simulink model "c00015M_harness"  (R2018a)
settings: Solver=FixedStepAuto  StartTime=0.0  StopTime=300  FixedStep=0.1  RelTol=1e-3
undefined symbols (not defined in the file): A1, hmax, PriorityTank, R1, R2, sigbuilder_block, TempThreshold
(part 3 of 33)

== system c00015M_harness/Eval21 ==
  In1 : Inport
  In3 : Inport  Port=2
  Constant2 : Constant
  Data Type Conversion : DataTypeConversion
  Data Type Conversion2 : DataTypeConversion
  Memory1 : Memory  InitialCondition=1
  Memory3 : Memory  InitialCondition=1
  MinMax : MinMax  Inputs=3
  MinMax1 : MinMax  Inputs=2
  MinMax3 : MinMax  Inputs=2
  ROOut1 : RelationalOperator  Operator===  OutDataTypeStr=boolean  RndMeth=Simplest
  ROOut3 : RelationalOperator  Operator===  OutDataTypeStr=boolean  RndMeth=Simplest
  Out1 : Outport
  wires:
  Data Type Conversion2/1 -> MinMax3/1
  Data Type Conversion/1 -> MinMax1/1
  MinMax1/1 -> Memory1/1, MinMax/1
  ROOut1/1 -> Data Type Conversion/1
  Memory3/1 -> MinMax3/2
  ROOut3/1 -> Data Type Conversion2/1
  MinMax3/1 -> Memory3/1, MinMax/3
  Memory1/1 -> MinMax1/2
  In1/1 -> ROOut1/1
  [out1] -> ROOut1/2
  In3/1 -> ROOut3/1
  [out3] -> ROOut3/2
  MinMax/1 -> Out1/1
  Constant2/1 -> MinMax/2

== system c00015M_harness/Eval22 ==
  In1 : Inport
  In3 : Inport  Port=2
  Constant2 : Constant
  Data Type Conversion : DataTypeConversion
  Data Type Conversion2 : DataTypeConversion
  Memory1 : Memory  InitialCondition=1
  Memory3 : Memory  InitialCondition=1
  MinMax : MinMax  Inputs=3
  MinMax1 : MinMax  Inputs=2
  MinMax3 : MinMax  Inputs=2
  ROOut1 : RelationalOperator  Operator===  OutDataTypeStr=boolean  RndMeth=Simplest
  ROOut3 : RelationalOperator  Operator===  OutDataTypeStr=boolean  RndMeth=Simplest
  Out1 : Outport
  wires:
  Data Type Conversion2/1 -> MinMax3/1
  Data Type Conversion/1 -> MinMax1/1
  MinMax1/1 -> Memory1/1, MinMax/1
  ROOut1/1 -> Data Type Conversion/1
  Memory3/1 -> MinMax3/2
  ROOut3/1 -> Data Type Conversion2/1
  MinMax3/1 -> Memory3/1, MinMax/3
  Memory1/1 -> MinMax1/2
  In1/1 -> ROOut1/1
  [out1] -> ROOut1/2
  In3/1 -> ROOut3/1
  [out3] -> ROOut3/2
  MinMax/1 -> Out1/1
  Constant2/1 -> MinMax/2

== system c00015M_harness/Eval220 ==
  In1 : Inport
  In3 : Inport  Port=2
  Constant2 : Constant
  Data Type Conversion : DataTypeConversion
  Data Type Conversion2 : DataTypeConversion
  Memory1 : Memory  InitialCondition=1
  Memory3 : Memory  InitialCondition=1
  MinMax : MinMax  Inputs=3
  MinMax1 : MinMax  Inputs=2
  MinMax3 : MinMax  Inputs=2
  ROOut1 : RelationalOperator  Operator===  OutDataTypeStr=boolean  RndMeth=Simplest
  ROOut3 : RelationalOperator  Operator===  OutDataTypeStr=boolean  RndMeth=Simplest
  Out1 : Outport
  wires:
  Data Type Conversion2/1 -> MinMax3/1
  Data Type Conversion/1 -> MinMax1/1
  MinMax1/1 -> Memory1/1, MinMax/1
  ROOut1/1 -> Data Type Conversion/1
  Memory3/1 -> MinMax3/2
  ROOut3/1 -> Data Type Conversion2/1
  MinMax3/1 -> Memory3/1, MinMax/3
  Memory1/1 -> MinMax1/2
  In1/1 -> ROOut1/1
  [out1] -> ROOut1/2
  In3/1 -> ROOut3/1
  [out3] -> ROOut3/2
  MinMax/1 -> Out1/1
  Constant2/1 -> MinMax/2

== system c00015M_harness/Eval221 ==
  In1 : Inport
  In3 : Inport  Port=2
  Constant2 : Constant
  Data Type Conversion : DataTypeConversion
  Data Type Conversion2 : DataTypeConversion
  Memory1 : Memory  InitialCondition=1
  Memory3 : Memory  InitialCondition=1
  MinMax : MinMax  Inputs=3
  MinMax1 : MinMax  Inputs=2
  MinMax3 : MinMax  Inputs=2
  ROOut1 : RelationalOperator  Operator===  OutDataTypeStr=boolean  RndMeth=Simplest
  ROOut3 : RelationalOperator  Operator===  OutDataTypeStr=boolean  RndMeth=Simplest
  Out1 : Outport
  wires:
  Data Type Conversion2/1 -> MinMax3/1
  Data Type Conversion/1 -> MinMax1/1
  MinMax1/1 -> Memory1/1, MinMax/1
  ROOut1/1 -> Data Type Conversion/1
  Memory3/1 -> MinMax3/2
  ROOut3/1 -> Data Type Conversion2/1
  MinMax3/1 -> Memory3/1, MinMax/3
  Memory1/1 -> MinMax1/2
  In1/1 -> ROOut1/1
  [out1] -> ROOut1/2
  In3/1 -> ROOut3/1
  [out3] -> ROOut3/2
  MinMax/1 -> Out1/1
  Constant2/1 -> MinMax/2

== system c00015M_harness/Eval222 ==
  In1 : Inport
  In3 : Inport  Port=2
  Constant2 : Constant
  Data Type Conversion : DataTypeConversion
  Data Type Conversion2 : DataTypeConversion
  Memory1 : Memory  InitialCondition=1
  Memory3 : Memory  InitialCondition=1
  MinMax : MinMax  Inputs=3
  MinMax1 : MinMax  Inputs=2
  MinMax3 : MinMax  Inputs=2
  ROOut1 : RelationalOperator  Operator===  OutDataTypeStr=boolean  RndMeth=Simplest
  ROOut3 : RelationalOperator  Operator===  OutDataTypeStr=boolean  RndMeth=Simplest
  Out1 : Outport
  wires:
  Data Type Conversion2/1 -> MinMax3/1
  Data Type Conversion/1 -> MinMax1/1
  MinMax1/1 -> Memory1/1, MinMax/1
  ROOut1/1 -> Data Type Conversion/1
  Memory3/1 -> MinMax3/2
  ROOut3/1 -> Data Type Conversion2/1
  MinMax3/1 -> Memory3/1, MinMax/3
  Memory1/1 -> MinMax1/2
  In1/1 -> ROOut1/1
  [out1] -> ROOut1/2
  In3/1 -> ROOut3/1
  [out3] -> ROOut3/2
  MinMax/1 -> Out1/1
  Constant2/1 -> MinMax/2

== system c00015M_harness/Eval223 ==
  In1 : Inport
  In3 : Inport  Port=2
  Constant2 : Constant
  Data Type Conversion : DataTypeConversion
  Data Type Conversion2 : DataTypeConversion
  Memory1 : Memory  InitialCondition=1
  Memory3 : Memory  InitialCondition=1
  MinMax : MinMax  Inputs=3
  MinMax1 : MinMax  Inputs=2
  MinMax3 : MinMax  Inputs=2
  ROOut1 : RelationalOperator  Operator===  OutDataTypeStr=boolean  RndMeth=Simplest
  ROOut3 : RelationalOperator  Operator===  OutDataTypeStr=boolean  RndMeth=Simplest
  Out1 : Outport
  wires:
  Data Type Conversion2/1 -> MinMax3/1
  Data Type Conversion/1 -> MinMax1/1
  MinMax1/1 -> Memory1/1, MinMax/1
  ROOut1/1 -> Data Type Conversion/1
  Memory3/1 -> MinMax3/2
  ROOut3/1 -> Data Type Conversion2/1
  MinMax3/1 -> Memory3/1, MinMax/3
  Memory1/1 -> MinMax1/2
  In1/1 -> ROOut1/1
  [out1] -> ROOut1/2
  In3/1 -> ROOut3/1
  [out3] -> ROOut3/2
  MinMax/1 -> Out1/1
  Constant2/1 -> MinMax/2

== system c00015M_harness/Eval224 ==
  In1 : Inport
  In3 : Inport  Port=2
  Constant2 : Constant
  Data Type Conversion : DataTypeConversion
  Data Type Conversion2 : DataTypeConversion
  Memory1 : Memory  InitialCondition=1
  Memory3 : Memory  InitialCondition=1
  MinMax : MinMax  Inputs=3
  MinMax1 : MinMax  Inputs=2
  MinMax3 : MinMax  Inputs=2
  ROOut1 : RelationalOperator  Operator===  OutDataTypeStr=boolean  RndMeth=Simplest
  ROOut3 : RelationalOperator  Operator===  OutDataTypeStr=boolean  RndMeth=Simplest
  Out1 : Outport
  wires:
  Data Type Conversion2/1 -> MinMax3/1
  Data Type Conversion/1 -> MinMax1/1
  MinMax1/1 -> Memory1/1, MinMax/1
  ROOut1/1 -> Data Type Conversion/1
  Memory3/1 -> MinMax3/2
  ROOut3/1 -> Data Type Conversion2/1
  MinMax3/1 -> Memory3/1, MinMax/3
  Memory1/1 -> MinMax1/2
  In1/1 -> ROOut1/1
  [out1] -> ROOut1/2
  In3/1 -> ROOut3/1
  [out3] -> ROOut3/2
  MinMax/1 -> Out1/1
  Constant2/1 -> MinMax/2

== system c00015M_harness/Eval225 ==
  In1 : Inport
  In3 : Inport  Port=2
  Constant2 : Constant
  Data Type Conversion : DataTypeConversion
  Data Type Conversion2 : DataTypeConversion
  Memory1 : Memory  InitialCondition=1
  Memory3 : Memory  InitialCondition=1
  MinMax : MinMax  Inputs=3
  MinMax1 : MinMax  Inputs=2
  MinMax3 : MinMax  Inputs=2
  ROOut1 : RelationalOperator  Operator===  OutDataTypeStr=boolean  RndMeth=Simplest
  ROOut3 : RelationalOperator  Operator===  OutDataTypeStr=boolean  RndMeth=Simplest
  Out1 : Outport
  wires:
  Data Type Conversion2/1 -> MinMax3/1
  Data Type Conversion/1 -> MinMax1/1
  MinMax1/1 -> Memory1/1, MinMax/1
  ROOut1/1 -> Data Type Conversion/1
  Memory3/1 -> MinMax3/2
  ROOut3/1 -> Data Type Conversion2/1
  MinMax3/1 -> Memory3/1, MinMax/3
  Memory1/1 -> MinMax1/2
  In1/1 -> ROOut1/1
  [out1] -> ROOut1/2
  In3/1 -> ROOut3/1
  [out3] -> ROOut3/2
  MinMax/1 -> Out1/1
  Constant2/1 -> MinMax/2

== system c00015M_harness/Eval226 ==
  In1 : Inport
  In3 : Inport  Port=2
  Constant2 : Constant
  Data Type Conversion : DataTypeConversion
  Data Type Conversion2 : DataTypeConversion
  Memory1 : Memory  InitialCondition=1
  Memory3 : Memory  InitialCondition=1
  MinMax : MinMax  Inputs=3
  MinMax1 : MinMax  Inputs=2
  MinMax3 : MinMax  Inputs=2
  ROOut1 : RelationalOperator  Operator===  OutDataTypeStr=boolean  RndMeth=Simplest
  ROOut3 : RelationalOperator  Operator===  OutDataTypeStr=boolean  RndMeth=Simplest
  Out1 : Outport
  wires:
  Data Type Conversion2/1 -> MinMax3/1
  Data Type Conversion/1 -> MinMax1/1
  MinMax1/1 -> Memory1/1, MinMax/1
  ROOut1/1 -> Data Type Conversion/1
  Memory3/1 -> MinMax3/2
  ROOut3/1 -> Data Type Conversion2/1
  MinMax3/1 -> Memory3/1, MinMax/3
  Memory1/1 -> MinMax1/2
  In1/1 -> ROOut1/1
  [out1] -> ROOut1/2
  In3/1 -> ROOut3/1
  [out3] -> ROOut3/2
  MinMax/1 -> Out1/1
  Constant2/1 -> MinMax/2

== system c00015M_harness/Eval227 ==
  In1 : Inport
  In3 : Inport  Port=2
  Constant2 : Constant
  Data Type Conversion : DataTypeConversion
  Data Type Conversion2 : DataTypeConversion
  Memory1 : Memory  InitialCondition=1
  Memory3 : Memory  InitialCondition=1
  MinMax : MinMax  Inputs=3
  MinMax1 : MinMax  Inputs=2
  MinMax3 : MinMax  Inputs=2
  ROOut1 : RelationalOperator  Operator===  OutDataTypeStr=boolean  RndMeth=Simplest
  ROOut3 : RelationalOperator  Operator===  OutDataTypeStr=boolean  RndMeth=Simplest
  Out1 : Outport
  wires:
  Data Type Conversion2/1 -> MinMax3/1
  Data Type Conversion/1 -> MinMax1/1
  MinMax1/1 -> Memory1/1, MinMax/1
  ROOut1/1 -> Data Type Conversion/1
  Memory3/1 -> MinMax3/2
  ROOut3/1 -> Data Type Conversion2/1
  MinMax3/1 -> Memory3/1, MinMax/3
  Memory1/1 -> MinMax1/2
  In1/1 -> ROOut1/1
  [out1] -> ROOut1/2
  In3/1 -> ROOut3/1
  [out3] -> ROOut3/2
  MinMax/1 -> Out1/1
  Constant2/1 -> MinMax/2

== system c00015M_harness/Eval228 ==
  In1 : Inport
  In3 : Inport  Port=2
  Constant2 : Constant
  Data Type Conversion : DataTypeConversion
  Data Type Conversion2 : DataTypeConversion
  Memory1 : Memory  InitialCondition=1
  Memory3 : Memory  InitialCondition=1
  MinMax : MinMax  Inputs=3
  MinMax1 : MinMax  Inputs=2
  MinMax3 : MinMax  Inputs=2
  ROOut1 : RelationalOperator  Operator===  OutDataTypeStr=boolean  RndMeth=Simplest
  ROOut3 : RelationalOperator  Operator===  OutDataTypeStr=boolean  RndMeth=Simplest
  Out1 : Outport
  wires:
  Data Type Conversion2/1 -> MinMax3/1
  Data Type Conversion/1 -> MinMax1/1
  MinMax1/1 -> Memory1/1, MinMax/1
  ROOut1/1 -> Data Type Conversion/1
  Memory3/1 -> MinMax3/2
  ROOut3/1 -> Data Type Conversion2/1
  MinMax3/1 -> Memory3/1, MinMax/3
  Memory1/1 -> MinMax1/2
  In1/1 -> ROOut1/1
  [out1] -> ROOut1/2
  In3/1 -> ROOut3/1
  [out3] -> ROOut3/2
  MinMax/1 -> Out1/1
  Constant2/1 -> MinMax/2

== system c00015M_harness/Eval229 ==
  In1 : Inport
  In3 : Inport  Port=2
  Constant2 : Constant
  Data Type Conversion : DataTypeConversion
  Data Type Conversion2 : DataTypeConversion
  Memory1 : Memory  InitialCondition=1
  Memory3 : Memory  InitialCondition=1
  MinMax : MinMax  Inputs=3
  MinMax1 : MinMax  Inputs=2
  MinMax3 : MinMax  Inputs=2
  ROOut1 : RelationalOperator  Operator===  OutDataTypeStr=boolean  RndMeth=Simplest
  ROOut3 : RelationalOperator  Operator===  OutDataTypeStr=boolean  RndMeth=Simplest
  Out1 : Outport
  wires:
  Data Type Conversion2/1 -> MinMax3/1
  Data Type Conversion/1 -> MinMax1/1
  MinMax1/1 -> Memory1/1, MinMax/1
  ROOut1/1 -> Data Type Conversion/1
  Memory3/1 -> MinMax3/2
  ROOut3/1 -> Data Type Conversion2/1
  MinMax3/1 -> Memory3/1, MinMax/3
  Memory1/1 -> MinMax1/2
  In1/1 -> ROOut1/1
  [out1] -> ROOut1/2
  In3/1 -> ROOut3/1
  [out3] -> ROOut3/2
  MinMax/1 -> Out1/1
  Constant2/1 -> MinMax/2

== system c00015M_harness/Eval23 ==
  In1 : Inport
  In3 : Inport  Port=2
  Constant2 : Constant
  Data Type Conversion : DataTypeConversion
  Data Type Conversion2 : DataTypeConversion
  Memory1 : Memory  InitialCondition=1
  Memory3 : Memory  InitialCondition=1
  MinMax : MinMax  Inputs=3
  MinMax1 : MinMax  Inputs=2
  MinMax3 : MinMax  Inputs=2
  ROOut1 : RelationalOperator  Operator===  OutDataTypeStr=boolean  RndMeth=Simplest
  ROOut3 : RelationalOperator  Operator===  OutDataTypeStr=boolean  RndMeth=Simplest
  Out1 : Outport
  wires:
  Data Type Conversion2/1 -> MinMax3/1
  Data Type Conversion/1 -> MinMax1/1
  MinMax1/1 -> Memory1/1, MinMax/1
  ROOut1/1 -> Data Type Conversion/1
  Memory3/1 -> MinMax3/2
  ROOut3/1 -> Data Type Conversion2/1
  MinMax3/1 -> Memory3/1, MinMax/3
  Memory1/1 -> MinMax1/2
  In1/1 -> ROOut1/1
  [out1] -> ROOut1/2
  In3/1 -> ROOut3/1
  [out3] -> ROOut3/2
  MinMax/1 -> Out1/1
  Constant2/1 -> MinMax/2

== system c00015M_harness/Eval230 ==
  In1 : Inport
  In3 : Inport  Port=2
  Constant2 : Constant
  Data Type Conversion : DataTypeConversion
  Data Type Conversion2 : DataTypeConversion
  Memory1 : Memory  InitialCondition=1
  Memory3 : Memory  InitialCondition=1
  MinMax : MinMax  Inputs=3
  MinMax1 : MinMax  Inputs=2
  MinMax3 : MinMax  Inputs=2
  ROOut1 : RelationalOperator  Operator===  OutDataTypeStr=boolean  RndMeth=Simplest
  ROOut3 : RelationalOperator  Operator===  OutDataTypeStr=boolean  RndMeth=Simplest
  Out1 : Outport
  wires:
  Data Type Conversion2/1 -> MinMax3/1
  Data Type Conversion/1 -> MinMax1/1
  MinMax1/1 -> Memory1/1, MinMax/1
  ROOut1/1 -> Data Type Conversion/1
  Memory3/1 -> MinMax3/2
  ROOut3/1 -> Data Type Conversion2/1
  MinMax3/1 -> Memory3/1, MinMax/3
  Memory1/1 -> MinMax1/2
  In1/1 -> ROOut1/1
  [out1] -> ROOut1/2
  In3/1 -> ROOut3/1
  [out3] -> ROOut3/2
  MinMax/1 -> Out1/1
  Constant2/1 -> MinMax/2

== system c00015M_harness/Eval231 ==
  In1 : Inport
  In3 : Inport  Port=2
  Constant2 : Constant
  Data Type Conversion : DataTypeConversion
  Data Type Conversion2 : DataTypeConversion
  Memory1 : Memory  InitialCondition=1
  Memory3 : Memory  InitialCondition=1
  MinMax : MinMax  Inputs=3
  MinMax1 : MinMax  Inputs=2
  MinMax3 : MinMax  Inputs=2
  ROOut1 : RelationalOperator  Operator===  OutDataTypeStr=boolean  RndMeth=Simplest
  ROOut3 : RelationalOperator  Operator===  OutDataTypeStr=boolean  RndMeth=Simplest
  Out1 : Outport
  wires:
  Data Type Conversion2/1 -> MinMax3/1
  Data Type Conversion/1 -> MinMax1/1
  MinMax1/1 -> Memory1/1, MinMax/1
  ROOut1/1 -> Data Type Conversion/1
  Memory3/1 -> MinMax3/2
  ROOut3/1 -> Data Type Conversion2/1
  MinMax3/1 -> Memory3/1, MinMax/3
  Memory1/1 -> MinMax1/2
  In1/1 -> ROOut1/1
  [out1] -> ROOut1/2
  In3/1 -> ROOut3/1
  [out3] -> ROOut3/2
  MinMax/1 -> Out1/1
  Constant2/1 -> MinMax/2

== system c00015M_harness/Eval232 ==
  In1 : Inport
  In3 : Inport  Port=2
  Constant2 : Constant
  Data Type Conversion : DataTypeConversion
  Data Type Conversion2 : DataTypeConversion
  Memory1 : Memory  InitialCondition=1
  Memory3 : Memory  InitialCondition=1
  MinMax : MinMax  Inputs=3
  MinMax1 : MinMax  Inputs=2
  MinMax3 : MinMax  Inputs=2
  ROOut1 : RelationalOperator  Operator===  OutDataTypeStr=boolean  RndMeth=Simplest
  ROOut3 : RelationalOperator  Operator===  OutDataTypeStr=boolean  RndMeth=Simplest
  Out1 : Outport
  wires:
  Data Type Conversion2/1 -> MinMax3/1
  Data Type Conversion/1 -> MinMax1/1
  MinMax1/1 -> Memory1/1, MinMax/1
  ROOut1/1 -> Data Type Conversion/1
  Memory3/1 -> MinMax3/2
  ROOut3/1 -> Data Type Conversion2/1
  MinMax3/1 -> Memory3/1, MinMax/3
  Memory1/1 -> MinMax1/2
  In1/1 -> ROOut1/1
  [out1] -> ROOut1/2
  In3/1 -> ROOut3/1
  [out3] -> ROOut3/2
  MinMax/1 -> Out1/1
  Constant2/1 -> MinMax/2

== system c00015M_harness/Eval233 ==
  In1 : Inport
  In3 : Inport  Port=2
  Constant2 : Constant
  Data Type Conversion : DataTypeConversion
  Data Type Conversion2 : DataTypeConversion
  Memory1 : Memory  InitialCondition=1
  Memory3 : Memory  InitialCondition=1
  MinMax : MinMax  Inputs=3
  MinMax1 : MinMax  Inputs=2
  MinMax3 : MinMax  Inputs=2
  ROOut1 : RelationalOperator  Operator===  OutDataTypeStr=boolean  RndMeth=Simplest
  ROOut3 : RelationalOperator  Operator===  OutDataTypeStr=boolean  RndMeth=Simplest
  Out1 : Outport
  wires:
  Data Type Conversion2/1 -> MinMax3/1
  Data Type Conversion/1 -> MinMax1/1
  MinMax1/1 -> Memory1/1, MinMax/1
  ROOut1/1 -> Data Type Conversion/1
  Memory3/1 -> MinMax3/2
  ROOut3/1 -> Data Type Conversion2/1
  MinMax3/1 -> Memory3/1, MinMax/3
  Memory1/1 -> MinMax1/2
  In1/1 -> ROOut1/1
  [out1] -> ROOut1/2
  In3/1 -> ROOut3/1
  [out3] -> ROOut3/2
  MinMax/1 -> Out1/1
  Constant2/1 -> MinMax/2

== system c00015M_harness/Eval234 ==
  In1 : Inport
  In3 : Inport  Port=2
  Constant2 : Constant
  Data Type Conversion : DataTypeConversion
  Data Type Conversion2 : DataTypeConversion
  Memory1 : Memory  InitialCondition=1
  Memory3 : Memory  InitialCondition=1
  MinMax : MinMax  Inputs=3
  MinMax1 : MinMax  Inputs=2
  MinMax3 : MinMax  Inputs=2
  ROOut1 : RelationalOperator  Operator===  OutDataTypeStr=boolean  RndMeth=Simplest
  ROOut3 : RelationalOperator  Operator===  OutDataTypeStr=boolean  RndMeth=Simplest
  Out1 : Outport
  wires:
  Data Type Conversion2/1 -> MinMax3/1
  Data Type Conversion/1 -> MinMax1/1
  MinMax1/1 -> Memory1/1, MinMax/1
  ROOut1/1 -> Data Type Conversion/1
  Memory3/1 -> MinMax3/2
  ROOut3/1 -> Data Type Conversion2/1
  MinMax3/1 -> Memory3/1, MinMax/3
  Memory1/1 -> MinMax1/2
  In1/1 -> ROOut1/1
  [out1] -> ROOut1/2
  In3/1 -> ROOut3/1
  [out3] -> ROOut3/2
  MinMax/1 -> Out1/1
  Constant2/1 -> MinMax/2

== system c00015M_harness/Eval235 ==
  In1 : Inport
  In3 : Inport  Port=2
  Constant2 : Constant
  Data Type Conversion : DataTypeConversion
  Data Type Conversion2 : DataTypeConversion
  Memory1 : Memory  InitialCondition=1
  Memory3 : Memory  InitialCondition=1
  MinMax : MinMax  Inputs=3
  MinMax1 : MinMax  Inputs=2
  MinMax3 : MinMax  Inputs=2
  ROOut1 : RelationalOperator  Operator===  OutDataTypeStr=boolean  RndMeth=Simplest
  ROOut3 : RelationalOperator  Operator===  OutDataTypeStr=boolean  RndMeth=Simplest
  Out1 : Outport
  wires:
  Data Type Conversion2/1 -> MinMax3/1
  Data Type Conversion/1 -> MinMax1/1
  MinMax1/1 -> Memory1/1, MinMax/1
  ROOut1/1 -> Data Type Conversion/1
  Memory3/1 -> MinMax3/2
  ROOut3/1 -> Data Type Conversion2/1
  MinMax3/1 -> Memory3/1, MinMax/3
  Memory1/1 -> MinMax1/2
  In1/1 -> ROOut1/1
  [out1] -> ROOut1/2
  In3/1 -> ROOut3/1
  [out3] -> ROOut3/2
  MinMax/1 -> Out1/1
  Constant2/1 -> MinMax/2

== system c00015M_harness/Eval236 ==
  In1 : Inport
  In3 : Inport  Port=2
  Constant2 : Constant
  Data Type Conversion : DataTypeConversion
  Data Type Conversion2 : DataTypeConversion
  Memory1 : Memory  InitialCondition=1
  Memory3 : Memory  InitialCondition=1
  MinMax : MinMax  Inputs=3
  MinMax1 : MinMax  Inputs=2
  MinMax3 : MinMax  Inputs=2
  ROOut1 : RelationalOperator  Operator===  OutDataTypeStr=boolean  RndMeth=Simplest
  ROOut3 : RelationalOperator  Operator===  OutDataTypeStr=boolean  RndMeth=Simplest
  Out1 : Outport
  wires:
  Data Type Conversion2/1 -> MinMax3/1
  Data Type Conversion/1 -> MinMax1/1
  MinMax1/1 -> Memory1/1, MinMax/1
  ROOut1/1 -> Data Type Conversion/1
  Memory3/1 -> MinMax3/2
  ROOut3/1 -> Data Type Conversion2/1
  MinMax3/1 -> Memory3/1, MinMax/3
  Memory1/1 -> MinMax1/2
  In1/1 -> ROOut1/1
  [out1] -> ROOut1/2
  In3/1 -> ROOut3/1
  [out3] -> ROOut3/2
  MinMax/1 -> Out1/1
  Constant2/1 -> MinMax/2

== system c00015M_harness/Eval237 ==
  In1 : Inport
  In3 : Inport  Port=2
  Constant2 : Constant
  Data Type Conversion : DataTypeConversion
  Data Type Conversion2 : DataTypeConversion
  Memory1 : Memory  InitialCondition=1
  Memory3 : Memory  InitialCondition=1
  MinMax : MinMax  Inputs=3
  MinMax1 : MinMax  Inputs=2
  MinMax3 : MinMax  Inputs=2
  ROOut1 : RelationalOperator  Operator===  OutDataTypeStr=boolean  RndMeth=Simplest
  ROOut3 : RelationalOperator  Operator===  OutDataTypeStr=boolean  RndMeth=Simplest
  Out1 : Outport
  wires:
  Data Type Conversion2/1 -> MinMax3/1
  Data Type Conversion/1 -> MinMax1/1
  MinMax1/1 -> Memory1/1, MinMax/1
  ROOut1/1 -> Data Type Conversion/1
  Memory3/1 -> MinMax3/2
  ROOut3/1 -> Data Type Conversion2/1
  MinMax3/1 -> Memory3/1, MinMax/3
  Memory1/1 -> MinMax1/2
  In1/1 -> ROOut1/1
  [out1] -> ROOut1/2
  In3/1 -> ROOut3/1
  [out3] -> ROOut3/2
  MinMax/1 -> Out1/1
  Constant2/1 -> MinMax/2

== system c00015M_harness/Eval238 ==
  In1 : Inport
  In3 : Inport  Port=2
  Constant2 : Constant
  Data Type Conversion : DataTypeConversion
  Data Type Conversion2 : DataTypeConversion
  Memory1 : Memory  InitialCondition=1
  Memory3 : Memory  InitialCondition=1
  MinMax : MinMax  Inputs=3
  MinMax1 : MinMax  Inputs=2
  MinMax3 : MinMax  Inputs=2
  ROOut1 : RelationalOperator  Operator===  OutDataTypeStr=boolean  RndMeth=Simplest
  ROOut3 : RelationalOperator  Operator===  OutDataTypeStr=boolean  RndMeth=Simplest
  Out1 : Outport
  wires:
  Data Type Conversion2/1 -> MinMax3/1
  Data Type Conversion/1 -> MinMax1/1
  MinMax1/1 -> Memory1/1, MinMax/1
  ROOut1/1 -> Data Type Conversion/1
  Memory3/1 -> MinMax3/2
  ROOut3/1 -> Data Type Conversion2/1
  MinMax3/1 -> Memory3/1, MinMax/3
  Memory1/1 -> MinMax1/2
  In1/1 -> ROOut1/1
  [out1] -> ROOut1/2
  In3/1 -> ROOut3/1
  [out3] -> ROOut3/2
  MinMax/1 -> Out1/1
  Constant2/1 -> MinMax/2

== system c00015M_harness/Eval239 ==
  In1 : Inport
  In3 : Inport  Port=2
  Constant2 : Constant
  Data Type Conversion : DataTypeConversion
  Data Type Conversion2 : DataTypeConversion
  Memory1 : Memory  InitialCondition=1
  Memory3 : Memory  InitialCondition=1
  MinMax : MinMax  Inputs=3
  MinMax1 : MinMax  Inputs=2
  MinMax3 : MinMax  Inputs=2
  ROOut1 : RelationalOperator  Operator===  OutDataTypeStr=boolean  RndMeth=Simplest
  ROOut3 : RelationalOperator  Operator===  OutDataTypeStr=boolean  RndMeth=Simplest
  Out1 : Outport
  wires:
  Data Type Conversion2/1 -> MinMax3/1
  Data Type Conversion/1 -> MinMax1/1
  MinMax1/1 -> Memory1/1, MinMax/1
  ROOut1/1 -> Data Type Conversion/1
  Memory3/1 -> MinMax3/2
  ROOut3/1 -> Data Type Conversion2/1
  MinMax3/1 -> Memory3/1, MinMax/3
  Memory1/1 -> MinMax1/2
  In1/1 -> ROOut1/1
  [out1] -> ROOut1/2
  In3/1 -> ROOut3/1
  [out3] -> ROOut3/2
  MinMax/1 -> Out1/1
  Constant2/1 -> MinMax/2

== system c00015M_harness/Eval24 ==
  In1 : Inport
  In3 : Inport  Port=2
  Constant2 : Constant
  Data Type Conversion : DataTypeConversion
  Data Type Conversion2 : DataTypeConversion
  Memory1 : Memory  InitialCondition=1
  Memory3 : Memory  InitialCondition=1
  MinMax : MinMax  Inputs=3
  MinMax1 : MinMax  Inputs=2
  MinMax3 : MinMax  Inputs=2
  ROOut1 : RelationalOperator  Operator===  OutDataTypeStr=boolean  RndMeth=Simplest
  ROOut3 : RelationalOperator  Operator===  OutDataTypeStr=boolean  RndMeth=Simplest
  Out1 : Outport
  wires:
  Data Type Conversion2/1 -> MinMax3/1
  Data Type Conversion/1 -> MinMax1/1
  MinMax1/1 -> Memory1/1, MinMax/1
  ROOut1/1 -> Data Type Conversion/1
  Memory3/1 -> MinMax3/2
  ROOut3/1 -> Data Type Conversion2/1
  MinMax3/1 -> Memory3/1, MinMax/3
  Memory1/1 -> MinMax1/2
  In1/1 -> ROOut1/1
  [out1] -> ROOut1/2
  In3/1 -> ROOut3/1
  [out3] -> ROOut3/2
  MinMax/1 -> Out1/1
  Constant2/1 -> MinMax/2

== system c00015M_harness/Eval240 ==
  In1 : Inport
  In3 : Inport  Port=2
  Constant2 : Constant
  Data Type Conversion : DataTypeConversion
  Data Type Conversion2 : DataTypeConversion
  Memory1 : Memory  InitialCondition=1
  Memory3 : Memory  InitialCondition=1
  MinMax : MinMax  Inputs=3
  MinMax1 : MinMax  Inputs=2
  MinMax3 : MinMax  Inputs=2
  ROOut1 : RelationalOperator  Operator===  OutDataTypeStr=boolean  RndMeth=Simplest
  ROOut3 : RelationalOperator  Operator===  OutDataTypeStr=boolean  RndMeth=Simplest
  Out1 : Outport
  wires:
  Data Type Conversion2/1 -> MinMax3/1
  Data Type Conversion/1 -> MinMax1/1
  MinMax1/1 -> Memory1/1, MinMax/1
  ROOut1/1 -> Data Type Conversion/1
  Memory3/1 -> MinMax3/2
  ROOut3/1 -> Data Type Conversion2/1
  MinMax3/1 -> Memory3/1, MinMax/3
  Memory1/1 -> MinMax1/2
  In1/1 -> ROOut1/1
  [out1] -> ROOut1/2
  In3/1 -> ROOut3/1
  [out3] -> ROOut3/2
  MinMax/1 -> Out1/1
  Constant2/1 -> MinMax/2

== system c00015M_harness/Eval241 ==
  In1 : Inport
  In3 : Inport  Port=2
  Constant2 : Constant
  Data Type Conversion : DataTypeConversion
  Data Type Conversion2 : DataTypeConversion
  Memory1 : Memory  InitialCondition=1
  Memory3 : Memory  InitialCondition=1
  MinMax : MinMax  Inputs=3
  MinMax1 : MinMax  Inputs=2
  MinMax3 : MinMax  Inputs=2
  ROOut1 : RelationalOperator  Operator===  OutDataTypeStr=boolean  RndMeth=Simplest
  ROOut3 : RelationalOperator  Operator===  OutDataTypeStr=boolean  RndMeth=Simplest
  Out1 : Outport
  wires:
  Data Type Conversion2/1 -> MinMax3/1
  Data Type Conversion/1 -> MinMax1/1
  MinMax1/1 -> Memory1/1, MinMax/1
  ROOut1/1 -> Data Type Conversion/1
  Memory3/1 -> MinMax3/2
  ROOut3/1 -> Data Type Conversion2/1
  MinMax3/1 -> Memory3/1, MinMax/3
  Memory1/1 -> MinMax1/2
  In1/1 -> ROOut1/1
  [out1] -> ROOut1/2
  In3/1 -> ROOut3/1
  [out3] -> ROOut3/2
  MinMax/1 -> Out1/1
  Constant2/1 -> MinMax/2

== system c00015M_harness/Eval242 ==
  In1 : Inport
  In3 : Inport  Port=2
  Constant2 : Constant
  Data Type Conversion : DataTypeConversion
  Data Type Conversion2 : DataTypeConversion
  Memory1 : Memory  InitialCondition=1
  Memory3 : Memory  InitialCondition=1
  MinMax : MinMax  Inputs=3
  MinMax1 : MinMax  Inputs=2
  MinMax3 : MinMax  Inputs=2
  ROOut1 : RelationalOperator  Operator===  OutDataTypeStr=boolean  RndMeth=Simplest
  ROOut3 : RelationalOperator  Operator===  OutDataTypeStr=boolean  RndMeth=Simplest
  Out1 : Outport
  wires:
  Data Type Conversion2/1 -> MinMax3/1
  Data Type Conversion/1 -> MinMax1/1
  MinMax1/1 -> Memory1/1, MinMax/1
  ROOut1/1 -> Data Type Conversion/1
  Memory3/1 -> MinMax3/2
  ROOut3/1 -> Data Type Conversion2/1
  MinMax3/1 -> Memory3/1, MinMax/3
  Memory1/1 -> MinMax1/2
  In1/1 -> ROOut1/1
  [out1] -> ROOut1/2
  In3/1 -> ROOut3/1
  [out3] -> ROOut3/2
  MinMax/1 -> Out1/1
  Constant2/1 -> MinMax/2

== system c00015M_harness/Eval243 ==
  In1 : Inport
  In3 : Inport  Port=2
  Constant2 : Constant
  Data Type Conversion : DataTypeConversion
  Data Type Conversion2 : DataTypeConversion
  Memory1 : Memory  InitialCondition=1
  Memory3 : Memory  InitialCondition=1
  MinMax : MinMax  Inputs=3
  MinMax1 : MinMax  Inputs=2
  MinMax3 : MinMax  Inputs=2
  ROOut1 : RelationalOperator  Operator===  OutDataTypeStr=boolean  RndMeth=Simplest
  ROOut3 : RelationalOperator  Operator===  OutDataTypeStr=boolean  RndMeth=Simplest
  Out1 : Outport
  wires:
  Data Type Conversion2/1 -> MinMax3/1
  Data Type Conversion/1 -> MinMax1/1
  MinMax1/1 -> Memory1/1, MinMax/1
  ROOut1/1 -> Data Type Conversion/1
  Memory3/1 -> MinMax3/2
  ROOut3/1 -> Data Type Conversion2/1
  MinMax3/1 -> Memory3/1, MinMax/3
  Memory1/1 -> MinMax1/2
  In1/1 -> ROOut1/1
  [out1] -> ROOut1/2
  In3/1 -> ROOut3/1
  [out3] -> ROOut3/2
  MinMax/1 -> Out1/1
  Constant2/1 -> MinMax/2

== system c00015M_harness/Eval244 ==
  In1 : Inport
  In3 : Inport  Port=2
  Constant2 : Constant
  Data Type Conversion : DataTypeConversion
  Data Type Conversion2 : DataTypeConversion
  Memory1 : Memory  InitialCondition=1
  Memory3 : Memory  InitialCondition=1
  MinMax : MinMax  Inputs=3
  MinMax1 : MinMax  Inputs=2
  MinMax3 : MinMax  Inputs=2
  ROOut1 : RelationalOperator  Operator===  OutDataTypeStr=boolean  RndMeth=Simplest
  ROOut3 : RelationalOperator  Operator===  OutDataTypeStr=boolean  RndMeth=Simplest
  Out1 : Outport
  wires:
  Data Type Conversion2/1 -> MinMax3/1
  Data Type Conversion/1 -> MinMax1/1
  MinMax1/1 -> Memory1/1, MinMax/1
  ROOut1/1 -> Data Type Conversion/1
  Memory3/1 -> MinMax3/2
  ROOut3/1 -> Data Type Conversion2/1
  MinMax3/1 -> Memory3/1, MinMax/3
  Memory1/1 -> MinMax1/2
  In1/1 -> ROOut1/1
  [out1] -> ROOut1/2
  In3/1 -> ROOut3/1
  [out3] -> ROOut3/2
  MinMax/1 -> Out1/1
  Constant2/1 -> MinMax/2

== system c00015M_harness/Eval245 ==
  In1 : Inport
  In3 : Inport  Port=2
  Constant2 : Constant
  Data Type Conversion : DataTypeConversion
  Data Type Conversion2 : DataTypeConversion
  Memory1 : Memory  InitialCondition=1
  Memory3 : Memory  InitialCondition=1
  MinMax : MinMax  Inputs=3
  MinMax1 : MinMax  Inputs=2
  MinMax3 : MinMax  Inputs=2
  ROOut1 : RelationalOperator  Operator===  OutDataTypeStr=boolean  RndMeth=Simplest
  ROOut3 : RelationalOperator  Operator===  OutDataTypeStr=boolean  RndMeth=Simplest
  Out1 : Outport
  wires:
  Data Type Conversion2/1 -> MinMax3/1
  Data Type Conversion/1 -> MinMax1/1
  MinMax1/1 -> Memory1/1, MinMax/1
  ROOut1/1 -> Data Type Conversion/1
  Memory3/1 -> MinMax3/2
  ROOut3/1 -> Data Type Conversion2/1
  MinMax3/1 -> Memory3/1, MinMax/3
  Memory1/1 -> MinMax1/2
  In1/1 -> ROOut1/1
  [out1] -> ROOut1/2
  In3/1 -> ROOut3/1
  [out3] -> ROOut3/2
  MinMax/1 -> Out1/1
  Constant2/1 -> MinMax/2

== system c00015M_harness/Eval25 ==
  In1 : Inport
  In3 : Inport  Port=2
  Constant2 : Constant
  Data Type Conversion : DataTypeConversion
  Data Type Conversion2 : DataTypeConversion
  Memory1 : Memory  InitialCondition=1
  Memory3 : Memory  InitialCondition=1
  MinMax : MinMax  Inputs=3
  MinMax1 : MinMax  Inputs=2
  MinMax3 : MinMax  Inputs=2
  ROOut1 : RelationalOperator  Operator===  OutDataTypeStr=boolean  RndMeth=Simplest
  ROOut3 : RelationalOperator  Operator===  OutDataTypeStr=boolean  RndMeth=Simplest
  Out1 : Outport
  wires:
  Data Type Conversion2/1 -> MinMax3/1
  Data Type Conversion/1 -> MinMax1/1
  MinMax1/1 -> Memory1/1, MinMax/1
  ROOut1/1 -> Data Type Conversion/1
  Memory3/1 -> MinMax3/2
  ROOut3/1 -> Data Type Conversion2/1
  MinMax3/1 -> Memory3/1, MinMax/3
  Memory1/1 -> MinMax1/2
  In1/1 -> ROOut1/1
  [out1] -> ROOut1/2
  In3/1 -> ROOut3/1
  [out3] -> ROOut3/2
  MinMax/1 -> Out1/1
  Constant2/1 -> MinMax/2

== system c00015M_harness/Eval26 ==
  In1 : Inport
  In3 : Inport  Port=2
  Constant2 : Constant
  Data Type Conversion : DataTypeConversion
  Data Type Conversion2 : DataTypeConversion
  Memory1 : Memory  InitialCondition=1
  Memory3 : Memory  InitialCondition=1
  MinMax : MinMax  Inputs=3
  MinMax1 : MinMax  Inputs=2
  MinMax3 : MinMax  Inputs=2
  ROOut1 : RelationalOperator  Operator===  OutDataTypeStr=boolean  RndMeth=Simplest
  ROOut3 : RelationalOperator  Operator===  OutDataTypeStr=boolean  RndMeth=Simplest
  Out1 : Outport
  wires:
  Data Type Conversion2/1 -> MinMax3/1
  Data Type Conversion/1 -> MinMax1/1
  MinMax1/1 -> Memory1/1, MinMax/1
  ROOut1/1 -> Data Type Conversion/1
  Memory3/1 -> MinMax3/2
  ROOut3/1 -> Data Type Conversion2/1
  MinMax3/1 -> Memory3/1, MinMax/3
  Memory1/1 -> MinMax1/2
  In1/1 -> ROOut1/1
  [out1] -> ROOut1/2
  In3/1 -> ROOut3/1
  [out3] -> ROOut3/2
  MinMax/1 -> Out1/1
  Constant2/1 -> MinMax/2

== system c00015M_harness/Eval27 ==
  In1 : Inport
  In3 : Inport  Port=2
  Constant2 : Constant
  Data Type Conversion : DataTypeConversion
  Data Type Conversion2 : DataTypeConversion
  Memory1 : Memory  InitialCondition=1
  Memory3 : Memory  InitialCondition=1
  MinMax : MinMax  Inputs=3
  MinMax1 : MinMax  Inputs=2
  MinMax3 : MinMax  Inputs=2
  ROOut1 : RelationalOperator  Operator===  OutDataTypeStr=boolean  RndMeth=Simplest
  ROOut3 : RelationalOperator  Operator===  OutDataTypeStr=boolean  RndMeth=Simplest
  Out1 : Outport
  wires:
  Data Type Conversion2/1 -> MinMax3/1
  Data Type Conversion/1 -> MinMax1/1
  MinMax1/1 -> Memory1/1, MinMax/1
  ROOut1/1 -> Data Type Conversion/1
  Memory3/1 -> MinMax3/2
  ROOut3/1 -> Data Type Conversion2/1
  MinMax3/1 -> Memory3/1, MinMax/3
  Memory1/1 -> MinMax1/2
  In1/1 -> ROOut1/1
  [out1] -> ROOut1/2
  In3/1 -> ROOut3/1
  [out3] -> ROOut3/2
  MinMax/1 -> Out1/1
  Constant2/1 -> MinMax/2

== system c00015M_harness/Eval28 ==
  In1 : Inport
  In3 : Inport  Port=2
  Constant2 : Constant
  Data Type Conversion : DataTypeConversion
  Data Type Conversion2 : DataTypeConversion
  Memory1 : Memory  InitialCondition=1
  Memory3 : Memory  InitialCondition=1
  MinMax : MinMax  Inputs=3
  MinMax1 : MinMax  Inputs=2
  MinMax3 : MinMax  Inputs=2
  ROOut1 : RelationalOperator  Operator===  OutDataTypeStr=boolean  RndMeth=Simplest
  ROOut3 : RelationalOperator  Operator===  OutDataTypeStr=boolean  RndMeth=Simplest
  Out1 : Outport
  wires:
  Data Type Conversion2/1 -> MinMax3/1
  Data Type Conversion/1 -> MinMax1/1
  MinMax1/1 -> Memory1/1, MinMax/1
  ROOut1/1 -> Data Type Conversion/1
  Memory3/1 -> MinMax3/2
  ROOut3/1 -> Data Type Conversion2/1
  MinMax3/1 -> Memory3/1, MinMax/3
  Memory1/1 -> MinMax1/2
  In1/1 -> ROOut1/1
  [out1] -> ROOut1/2
  In3/1 -> ROOut3/1
  [out3] -> ROOut3/2
  MinMax/1 -> Out1/1
  Constant2/1 -> MinMax/2

== system c00015M_harness/Eval29 ==
  In1 : Inport
  In3 : Inport  Port=2
  Constant2 : Constant
  Data Type Conversion : DataTypeConversion
  Data Type Conversion2 : DataTypeConversion
  Memory1 : Memory  InitialCondition=1
  Memory3 : Memory  InitialCondition=1
  MinMax : MinMax  Inputs=3
  MinMax1 : MinMax  Inputs=2
  MinMax3 : MinMax  Inputs=2
  ROOut1 : RelationalOperator  Operator===  OutDataTypeStr=boolean  RndMeth=Simplest
  ROOut3 : RelationalOperator  Operator===  OutDataTypeStr=boolean  RndMeth=Simplest
  Out1 : Outport
  wires:
  Data Type Conversion2/1 -> MinMax3/1
  Data Type Conversion/1 -> MinMax1/1
  MinMax1/1 -> Memory1/1, MinMax/1
  ROOut1/1 -> Data Type Conversion/1
  Memory3/1 -> MinMax3/2
  ROOut3/1 -> Data Type Conversion2/1
  MinMax3/1 -> Memory3/1, MinMax/3
  Memory1/1 -> MinMax1/2
  In1/1 -> ROOut1/1
  [out1] -> ROOut1/2
  In3/1 -> ROOut3/1
  [out3] -> ROOut3/2
  MinMax/1 -> Out1/1
  Constant2/1 -> MinMax/2

== system c00015M_harness/Eval3 ==
  In1 : Inport
  In3 : Inport  Port=2
  Constant2 : Constant
  Data Type Conversion : DataTypeConversion
  Data Type Conversion2 : DataTypeConversion
  Memory1 : Memory  InitialCondition=1
  Memory3 : Memory  InitialCondition=1
  MinMax : MinMax  Inputs=3
  MinMax1 : MinMax  Inputs=2
  MinMax3 : MinMax  Inputs=2
  ROOut1 : RelationalOperator  Operator===  OutDataTypeStr=boolean  RndMeth=Simplest
  ROOut3 : RelationalOperator  Operator===  OutDataTypeStr=boolean  RndMeth=Simplest
  Out1 : Outport
  wires:
  Data Type Conversion2/1 -> MinMax3/1
  Data Type Conversion/1 -> MinMax1/1
  MinMax1/1 -> Memory1/1, MinMax/1
  ROOut1/1 -> Data Type Conversion/1
  Memory3/1 -> MinMax3/2
  ROOut3/1 -> Data Type Conversion2/1
  MinMax3/1 -> Memory3/1, MinMax/3
  Memory1/1 -> MinMax1/2
  In1/1 -> ROOut1/1
  [out1] -> ROOut1/2
  In3/1 -> ROOut3/1
  [out3] -> ROOut3/2
  MinMax/1 -> Out1/1
  Constant2/1 -> MinMax/2

== system c00015M_harness/Eval30 ==
  In1 : Inport
  In3 : Inport  Port=2
  Constant2 : Constant
  Data Type Conversion : DataTypeConversion
  Data Type Conversion2 : DataTypeConversion
  Memory1 : Memory  InitialCondition=1
  Memory3 : Memory  InitialCondition=1
  MinMax : MinMax  Inputs=3
  MinMax1 : MinMax  Inputs=2
  MinMax3 : MinMax  Inputs=2
  ROOut1 : RelationalOperator  Operator===  OutDataTypeStr=boolean  RndMeth=Simplest
  ROOut3 : RelationalOperator  Operator===  OutDataTypeStr=boolean  RndMeth=Simplest
  Out1 : Outport
  wires:
  Data Type Conversion2/1 -> MinMax3/1
  Data Type Conversion/1 -> MinMax1/1
  MinMax1/1 -> Memory1/1, MinMax/1
  ROOut1/1 -> Data Type Conversion/1
  Memory3/1 -> MinMax3/2
  ROOut3/1 -> Data Type Conversion2/1
  MinMax3/1 -> Memory3/1, MinMax/3
  Memory1/1 -> MinMax1/2
  In1/1 -> ROOut1/1
  [out1] -> ROOut1/2
  In3/1 -> ROOut3/1
  [out3] -> ROOut3/2
  MinMax/1 -> Out1/1
  Constant2/1 -> MinMax/2

== system c00015M_harness/Eval31 ==
  In1 : Inport
  In3 : Inport  Port=2
  Constant2 : Constant
  Data Type Conversion : DataTypeConversion
  Data Type Conversion2 : DataTypeConversion
  Memory1 : Memory  InitialCondition=1
  Memory3 : Memory  InitialCondition=1
  MinMax : MinMax  Inputs=3
  MinMax1 : MinMax  Inputs=2
  MinMax3 : MinMax  Inputs=2
  ROOut1 : RelationalOperator  Operator===  OutDataTypeStr=boolean  RndMeth=Simplest
  ROOut3 : RelationalOperator  Operator===  OutDataTypeStr=boolean  RndMeth=Simplest
  Out1 : Outport
  wires:
  Data Type Conversion2/1 -> MinMax3/1
  Data Type Conversion/1 -> MinMax1/1
  MinMax1/1 -> Memory1/1, MinMax/1
  ROOut1/1 -> Data Type Conversion/1
  Memory3/1 -> MinMax3/2
  ROOut3/1 -> Data Type Conversion2/1
  MinMax3/1 -> Memory3/1, MinMax/3
  Memory1/1 -> MinMax1/2
  In1/1 -> ROOut1/1
  [out1] -> ROOut1/2
  In3/1 -> ROOut3/1
  [out3] -> ROOut3/2
  MinMax/1 -> Out1/1
  Constant2/1 -> MinMax/2

== system c00015M_harness/Eval32 ==
  In1 : Inport
  In3 : Inport  Port=2
  Constant2 : Constant
  Data Type Conversion : DataTypeConversion
  Data Type Conversion2 : DataTypeConversion
  Memory1 : Memory  InitialCondition=1
  Memory3 : Memory  InitialCondition=1
  MinMax : MinMax  Inputs=3
  MinMax1 : MinMax  Inputs=2
  MinMax3 : MinMax  Inputs=2
  ROOut1 : RelationalOperator  Operator===  OutDataTypeStr=boolean  RndMeth=Simplest
  ROOut3 : RelationalOperator  Operator===  OutDataTypeStr=boolean  RndMeth=Simplest
  Out1 : Outport
  wires:
  Data Type Conversion2/1 -> MinMax3/1
  Data Type Conversion/1 -> MinMax1/1
  MinMax1/1 -> Memory1/1, MinMax/1
  ROOut1/1 -> Data Type Conversion/1
  Memory3/1 -> MinMax3/2
  ROOut3/1 -> Data Type Conversion2/1
  MinMax3/1 -> Memory3/1, MinMax/3
  Memory1/1 -> MinMax1/2
  In1/1 -> ROOut1/1
  [out1] -> ROOut1/2
  In3/1 -> ROOut3/1
  [out3] -> ROOut3/2
  MinMax/1 -> Out1/1
  Constant2/1 -> MinMax/2

== system c00015M_harness/Eval33 ==
  In1 : Inport
  In3 : Inport  Port=2
  Constant2 : Constant
  Data Type Conversion : DataTypeConversion
  Data Type Conversion2 : DataTypeConversion
  Memory1 : Memory  InitialCondition=1
  Memory3 : Memory  InitialCondition=1
  MinMax : MinMax  Inputs=3
  MinMax1 : MinMax  Inputs=2
  MinMax3 : MinMax  Inputs=2
  ROOut1 : RelationalOperator  Operator===  OutDataTypeStr=boolean  RndMeth=Simplest
  ROOut3 : RelationalOperator  Operator===  OutDataTypeStr=boolean  RndMeth=Simplest
  Out1 : Outport
  wires:
  Data Type Conversion2/1 -> MinMax3/1
  Data Type Conversion/1 -> MinMax1/1
  MinMax1/1 -> Memory1/1, MinMax/1
  ROOut1/1 -> Data Type Conversion/1
  Memory3/1 -> MinMax3/2
  ROOut3/1 -> Data Type Conversion2/1
  MinMax3/1 -> Memory3/1, MinMax/3
  Memory1/1 -> MinMax1/2
  In1/1 -> ROOut1/1
  [out1] -> ROOut1/2
  In3/1 -> ROOut3/1
  [out3] -> ROOut3/2
  MinMax/1 -> Out1/1
  Constant2/1 -> MinMax/2

== system c00015M_harness/Eval34 ==
  In1 : Inport
  In3 : Inport  Port=2
  Constant2 : Constant
  Data Type Conversion : DataTypeConversion
  Data Type Conversion2 : DataTypeConversion
  Memory1 : Memory  InitialCondition=1
  Memory3 : Memory  InitialCondition=1
  MinMax : MinMax  Inputs=3
  MinMax1 : MinMax  Inputs=2
  MinMax3 : MinMax  Inputs=2
  ROOut1 : RelationalOperator  Operator===  OutDataTypeStr=boolean  RndMeth=Simplest
  ROOut3 : RelationalOperator  Operator===  OutDataTypeStr=boolean  RndMeth=Simplest
  Out1 : Outport
  wires:
  Data Type Conversion2/1 -> MinMax3/1
  Data Type Conversion/1 -> MinMax1/1
  MinMax1/1 -> Memory1/1, MinMax/1
  ROOut1/1 -> Data Type Conversion/1
  Memory3/1 -> MinMax3/2
  ROOut3/1 -> Data Type Conversion2/1
  MinMax3/1 -> Memory3/1, MinMax/3
  Memory1/1 -> MinMax1/2
  In1/1 -> ROOut1/1
  [out1] -> ROOut1/2
  In3/1 -> ROOut3/1
  [out3] -> ROOut3/2
  MinMax/1 -> Out1/1
  Constant2/1 -> MinMax/2

== system c00015M_harness/Eval4 ==
  In1 : Inport
  In3 : Inport  Port=2
  Constant2 : Constant
  Data Type Conversion : DataTypeConversion
  Data Type Conversion2 : DataTypeConversion
  Memory1 : Memory  InitialCondition=1
  Memory3 : Memory  InitialCondition=1
  MinMax : MinMax  Inputs=3
  MinMax1 : MinMax  Inputs=2
  MinMax3 : MinMax  Inputs=2
  ROOut1 : RelationalOperator  Operator===  OutDataTypeStr=boolean  RndMeth=Simplest
  ROOut3 : RelationalOperator  Operator===  OutDataTypeStr=boolean  RndMeth=Simplest
  Out1 : Outport
  wires:
  Data Type Conversion2/1 -> MinMax3/1
  Data Type Conversion/1 -> MinMax1/1
  MinMax1/1 -> Memory1/1, MinMax/1
  ROOut1/1 -> Data Type Conversion/1
  Memory3/1 -> MinMax3/2
  ROOut3/1 -> Data Type Conversion2/1
  MinMax3/1 -> Memory3/1, MinMax/3
  Memory1/1 -> MinMax1/2
  In1/1 -> ROOut1/1
  [out1] -> ROOut1/2
  In3/1 -> ROOut3/1
  [out3] -> ROOut3/2
  MinMax/1 -> Out1/1
  Constant2/1 -> MinMax/2

== system c00015M_harness/Eval5 ==
  In1 : Inport
  In3 : Inport  Port=2
  Constant2 : Constant
  Data Type Conversion : DataTypeConversion
  Data Type Conversion2 : DataTypeConversion
  Memory1 : Memory  InitialCondition=1
  Memory3 : Memory  InitialCondition=1
  MinMax : MinMax  Inputs=3
  MinMax1 : MinMax  Inputs=2
  MinMax3 : MinMax  Inputs=2
  ROOut1 : RelationalOperator  Operator===  OutDataTypeStr=boolean  RndMeth=Simplest
  ROOut3 : RelationalOperator  Operator===  OutDataTypeStr=boolean  RndMeth=Simplest
  Out1 : Outport
  wires:
  Data Type Conversion2/1 -> MinMax3/1
  Data Type Conversion/1 -> MinMax1/1
  MinMax1/1 -> Memory1/1, MinMax/1
  ROOut1/1 -> Data Type Conversion/1
  Memory3/1 -> MinMax3/2
  ROOut3/1 -> Data Type Conversion2/1
  MinMax3/1 -> Memory3/1, MinMax/3
  Memory1/1 -> MinMax1/2
  In1/1 -> ROOut1/1
  [out1] -> ROOut1/2
  In3/1 -> ROOut3/1
  [out3] -> ROOut3/2
  MinMax/1 -> Out1/1
  Constant2/1 -> MinMax/2

== system c00015M_harness/Eval56 ==
  In1 : Inport
  In3 : Inport  Port=2
  Constant2 : Constant
  Data Type Conversion : DataTypeConversion
  Data Type Conversion2 : DataTypeConversion
  Memory1 : Memory  InitialCondition=1
  Memory3 : Memory  InitialCondition=1
  MinMax : MinMax  Inputs=3
  MinMax1 : MinMax  Inputs=2
  MinMax3 : MinMax  Inputs=2
  ROOut1 : RelationalOperator  Operator===  OutDataTypeStr=boolean  RndMeth=Simplest
  ROOut3 : RelationalOperator  Operator===  OutDataTypeStr=boolean  RndMeth=Simplest
  Out1 : Outport
  wires:
  Data Type Conversion2/1 -> MinMax3/1
  Data Type Conversion/1 -> MinMax1/1
  MinMax1/1 -> Memory1/1, MinMax/1
  ROOut1/1 -> Data Type Conversion/1
  Memory3/1 -> MinMax3/2
  ROOut3/1 -> Data Type Conversion2/1
  MinMax3/1 -> Memory3/1, MinMax/3
  Memory1/1 -> MinMax1/2
  In1/1 -> ROOut1/1
  [out1] -> ROOut1/2
  In3/1 -> ROOut3/1
  [out3] -> ROOut3/2
  MinMax/1 -> Out1/1
  Constant2/1 -> MinMax/2

== system c00015M_harness/Eval57 ==
  In1 : Inport
  In3 : Inport  Port=2
  Constant2 : Constant
  Data Type Conversion : DataTypeConversion
  Data Type Conversion2 : DataTypeConversion
  Memory1 : Memory  InitialCondition=1
  Memory3 : Memory  InitialCondition=1
  MinMax : MinMax  Inputs=3
  MinMax1 : MinMax  Inputs=2
  MinMax3 : MinMax  Inputs=2
  ROOut1 : RelationalOperator  Operator===  OutDataTypeStr=boolean  RndMeth=Simplest
  ROOut3 : RelationalOperator  Operator===  OutDataTypeStr=boolean  RndMeth=Simplest
  Out1 : Outport
  wires:
  Data Type Conversion2/1 -> MinMax3/1
  Data Type Conversion/1 -> MinMax1/1
  MinMax1/1 -> Memory1/1, MinMax/1
  ROOut1/1 -> Data Type Conversion/1
  Memory3/1 -> MinMax3/2
  ROOut3/1 -> Data Type Conversion2/1
  MinMax3/1 -> Memory3/1, MinMax/3
  Memory1/1 -> MinMax1/2
  In1/1 -> ROOut1/1
  [out1] -> ROOut1/2
  In3/1 -> ROOut3/1
  [out3] -> ROOut3/2
  MinMax/1 -> Out1/1
  Constant2/1 -> MinMax/2

== system c00015M_harness/Eval58 ==
  In1 : Inport
  In3 : Inport  Port=2
  Constant2 : Constant
  Data Type Conversion : DataTypeConversion
  Data Type Conversion2 : DataTypeConversion
  Memory1 : Memory  InitialCondition=1
  Memory3 : Memory  InitialCondition=1
  MinMax : MinMax  Inputs=3
  MinMax1 : MinMax  Inputs=2
  MinMax3 : MinMax  Inputs=2
  ROOut1 : RelationalOperator  Operator===  OutDataTypeStr=boolean  RndMeth=Simplest
  ROOut3 : RelationalOperator  Operator===  OutDataTypeStr=boolean  RndMeth=Simplest
  Out1 : Outport
  wires:
  Data Type Conversion2/1 -> MinMax3/1
  Data Type Conversion/1 -> MinMax1/1
  MinMax1/1 -> Memory1/1, MinMax/1
  ROOut1/1 -> Data Type Conversion/1
  Memory3/1 -> MinMax3/2
  ROOut3/1 -> Data Type Conversion2/1
  MinMax3/1 -> Memory3/1, MinMax/3
  Memory1/1 -> MinMax1/2
  In1/1 -> ROOut1/1
  [out1] -> ROOut1/2
  In3/1 -> ROOut3/1
  [out3] -> ROOut3/2
  MinMax/1 -> Out1/1
  Constant2/1 -> MinMax/2

== system c00015M_harness/Eval59 ==
  In1 : Inport
  In3 : Inport  Port=2
  Constant2 : Constant
  Data Type Conversion : DataTypeConversion
  Data Type Conversion2 : DataTypeConversion
  Memory1 : Memory  InitialCondition=1
  Memory3 : Memory  InitialCondition=1
  MinMax : MinMax  Inputs=3
  MinMax1 : MinMax  Inputs=2
  MinMax3 : MinMax  Inputs=2
  ROOut1 : RelationalOperator  Operator===  OutDataTypeStr=boolean  RndMeth=Simplest
  ROOut3 : RelationalOperator  Operator===  OutDataTypeStr=boolean  RndMeth=Simplest
  Out1 : Outport
  wires:
  Data Type Conversion2/1 -> MinMax3/1
  Data Type Conversion/1 -> MinMax1/1
  MinMax1/1 -> Memory1/1, MinMax/1
  ROOut1/1 -> Data Type Conversion/1
  Memory3/1 -> MinMax3/2
  ROOut3/1 -> Data Type Conversion2/1
  MinMax3/1 -> Memory3/1, MinMax/3
  Memory1/1 -> MinMax1/2
  In1/1 -> ROOut1/1
  [out1] -> ROOut1/2
  In3/1 -> ROOut3/1
  [out3] -> ROOut3/2
  MinMax/1 -> Out1/1
  Constant2/1 -> MinMax/2

== system c00015M_harness/Eval6 ==
  In1 : Inport
  In3 : Inport  Port=2
  Constant2 : Constant
  Data Type Conversion : DataTypeConversion
  Data Type Conversion2 : DataTypeConversion
  Memory1 : Memory  InitialCondition=1
  Memory3 : Memory  InitialCondition=1
  MinMax : MinMax  Inputs=3
  MinMax1 : MinMax  Inputs=2
  MinMax3 : MinMax  Inputs=2
  ROOut1 : RelationalOperator  Operator===  OutDataTypeStr=boolean  RndMeth=Simplest
  ROOut3 : RelationalOperator  Operator===  OutDataTypeStr=boolean  RndMeth=Simplest
  Out1 : Outport
  wires:
  Data Type Conversion2/1 -> MinMax3/1
  Data Type Conversion/1 -> MinMax1/1
  MinMax1/1 -> Memory1/1, MinMax/1
  ROOut1/1 -> Data Type Conversion/1
  Memory3/1 -> MinMax3/2
  ROOut3/1 -> Data Type Conversion2/1
  MinMax3/1 -> Memory3/1, MinMax/3
  Memory1/1 -> MinMax1/2
  In1/1 -> ROOut1/1
  [out1] -> ROOut1/2
  In3/1 -> ROOut3/1
  [out3] -> ROOut3/2
  MinMax/1 -> Out1/1
  Constant2/1 -> MinMax/2

== system c00015M_harness/Eval60 ==
  In1 : Inport
  In3 : Inport  Port=2
  Constant2 : Constant
  Data Type Conversion : DataTypeConversion
  Data Type Conversion2 : DataTypeConversion
  Memory1 : Memory  InitialCondition=1
  Memory3 : Memory  InitialCondition=1
  MinMax : MinMax  Inputs=3
  MinMax1 : MinMax  Inputs=2
  MinMax3 : MinMax  Inputs=2
  ROOut1 : RelationalOperator  Operator===  OutDataTypeStr=boolean  RndMeth=Simplest
  ROOut3 : RelationalOperator  Operator===  OutDataTypeStr=boolean  RndMeth=Simplest
  Out1 : Outport
  wires:
  Data Type Conversion2/1 -> MinMax3/1
  Data Type Conversion/1 -> MinMax1/1
  MinMax1/1 -> Memory1/1, MinMax/1
  ROOut1/1 -> Data Type Conversion/1
  Memory3/1 -> MinMax3/2
  ROOut3/1 -> Data Type Conversion2/1
  MinMax3/1 -> Memory3/1, MinMax/3
  Memory1/1 -> MinMax1/2
  In1/1 -> ROOut1/1
  [out1] -> ROOut1/2
  In3/1 -> ROOut3/1
  [out3] -> ROOut3/2
  MinMax/1 -> Out1/1
  Constant2/1 -> MinMax/2

== system c00015M_harness/Eval61 ==
  In1 : Inport
  In3 : Inport  Port=2
  Constant2 : Constant
  Data Type Conversion : DataTypeConversion
  Data Type Conversion2 : DataTypeConversion
  Memory1 : Memory  InitialCondition=1
  Memory3 : Memory  InitialCondition=1
  MinMax : MinMax  Inputs=3
  MinMax1 : MinMax  Inputs=2
  MinMax3 : MinMax  Inputs=2
  ROOut1 : RelationalOperator  Operator===  OutDataTypeStr=boolean  RndMeth=Simplest
  ROOut3 : RelationalOperator  Operator===  OutDataTypeStr=boolean  RndMeth=Simplest
  Out1 : Outport
  wires:
  Data Type Conversion2/1 -> MinMax3/1
  Data Type Conversion/1 -> MinMax1/1
  MinMax1/1 -> Memory1/1, MinMax/1
  ROOut1/1 -> Data Type Conversion/1
  Memory3/1 -> MinMax3/2
  ROOut3/1 -> Data Type Conversion2/1
  MinMax3/1 -> Memory3/1, MinMax/3
  Memory1/1 -> MinMax1/2
  In1/1 -> ROOut1/1
  [out1] -> ROOut1/2
  In3/1 -> ROOut3/1
  [out3] -> ROOut3/2
  MinMax/1 -> Out1/1
  Constant2/1 -> MinMax/2

== system c00015M_harness/Eval62 ==
  In1 : Inport
  In3 : Inport  Port=2
  Constant2 : Constant
  Data Type Conversion : DataTypeConversion
  Data Type Conversion2 : DataTypeConversion
  Memory1 : Memory  InitialCondition=1
  Memory3 : Memory  InitialCondition=1
  MinMax : MinMax  Inputs=3
  MinMax1 : MinMax  Inputs=2
  MinMax3 : MinMax  Inputs=2
  ROOut1 : RelationalOperator  Operator===  OutDataTypeStr=boolean  RndMeth=Simplest
  ROOut3 : RelationalOperator  Operator===  OutDataTypeStr=boolean  RndMeth=Simplest
  Out1 : Outport
  wires:
  Data Type Conversion2/1 -> MinMax3/1
  Data Type Conversion/1 -> MinMax1/1
  MinMax1/1 -> Memory1/1, MinMax/1
  ROOut1/1 -> Data Type Conversion/1
  Memory3/1 -> MinMax3/2
  ROOut3/1 -> Data Type Conversion2/1
  MinMax3/1 -> Memory3/1, MinMax/3
  Memory1/1 -> MinMax1/2
  In1/1 -> ROOut1/1
  [out1] -> ROOut1/2
  In3/1 -> ROOut3/1
  [out3] -> ROOut3/2
  MinMax/1 -> Out1/1
  Constant2/1 -> MinMax/2

== system c00015M_harness/Eval63 ==
  In1 : Inport
  In3 : Inport  Port=2
  Constant2 : Constant
  Data Type Conversion : DataTypeConversion
  Data Type Conversion2 : DataTypeConversion
  Memory1 : Memory  InitialCondition=1
  Memory3 : Memory  InitialCondition=1
  MinMax : MinMax  Inputs=3
  MinMax1 : MinMax  Inputs=2
  MinMax3 : MinMax  Inputs=2
  ROOut1 : RelationalOperator  Operator===  OutDataTypeStr=boolean  RndMeth=Simplest
  ROOut3 : RelationalOperator  Operator===  OutDataTypeStr=boolean  RndMeth=Simplest
  Out1 : Outport
  wires:
  Data Type Conversion2/1 -> MinMax3/1
  Data Type Conversion/1 -> MinMax1/1
  MinMax1/1 -> Memory1/1, MinMax/1
  ROOut1/1 -> Data Type Conversion/1
  Memory3/1 -> MinMax3/2
  ROOut3/1 -> Data Type Conversion2/1
  MinMax3/1 -> Memory3/1, MinMax/3
  Memory1/1 -> MinMax1/2
  In1/1 -> ROOut1/1
  [out1] -> ROOut1/2
  In3/1 -> ROOut3/1
  [out3] -> ROOut3/2
  MinMax/1 -> Out1/1
  Constant2/1 -> MinMax/2
